simulink model "sixth_harmonic"  (R2013a)
settings: Solver=ode4  StartTime=0.0  StopTime=0.1  FixedStep=Ts  RelTol=1e-3
values from neighbouring files (symbols this model uses):
  Ip1 = Iline_fund*sqrt(2)    [acemp_sixth.m]    (also in immd_simulation_base.m)
  Ip3 = Iline_three*sqrt(2)    [acemp_sixth.m]    (also in immd_simulation_base.m)
  Lload = Xload/wout_fund    [acemp_sixth.m]    (also in immd_base_varyingmod.m = Xload/wout; immd_design_elen.m = Xload/wout; immd_efficiency.m = Xload/wout; immd_simulation_base.m)
  ma1 = 0.8    [acemp_sixth.m]    (also in immd_simulation_base.m)
  ma3 = 0.3    [acemp_sixth.m]    (also in immd_simulation_base.m)
  Rload = Zload*pf    [acemp_sixth.m]    (also in immd_base_varyingmod.m; immd_design_elen.m; immd_efficiency.m; immd_simulation_base.m)
  Ts = 1e-6    (= 1e-06)    [acemp_sixth.m]    (also in immd_base_varyingmod.m = 1e-05; immd_design_elen.m; immd_efficiency.m; immd_simulation_base.m)
  Vdc = (3/pi)*Vs_ll*sqrt(2)    [IMMD_design_tool_v01.m]    (also in IMMD_design_tool_v02.m; acemp_sixth.m = 400; immd_base_varyingmod.m = 400; immd_capacitor_rms_current.m = 400)
  Vp1 = ma1*Vdc/2    (= 160)    [acemp_sixth.m]    (also in immd_simulation_base.m)
  Vp3 = ma3*Vdc/2    (= 60)    [acemp_sixth.m]    (also in immd_simulation_base.m)
  wout_fund = 2*pi*fout_fund    (= 314.159265359)    [acemp_sixth.m]    (also in immd_simulation_base.m)
  wout_three = 2*pi*fout_three    (= 942.477796077)    [acemp_sixth.m]    (also in immd_simulation_base.m)
libraries: powerlib x32, powerlib_meascontrol x14
settings Model: Creator=ugurm  LastModifiedBy=ugurm

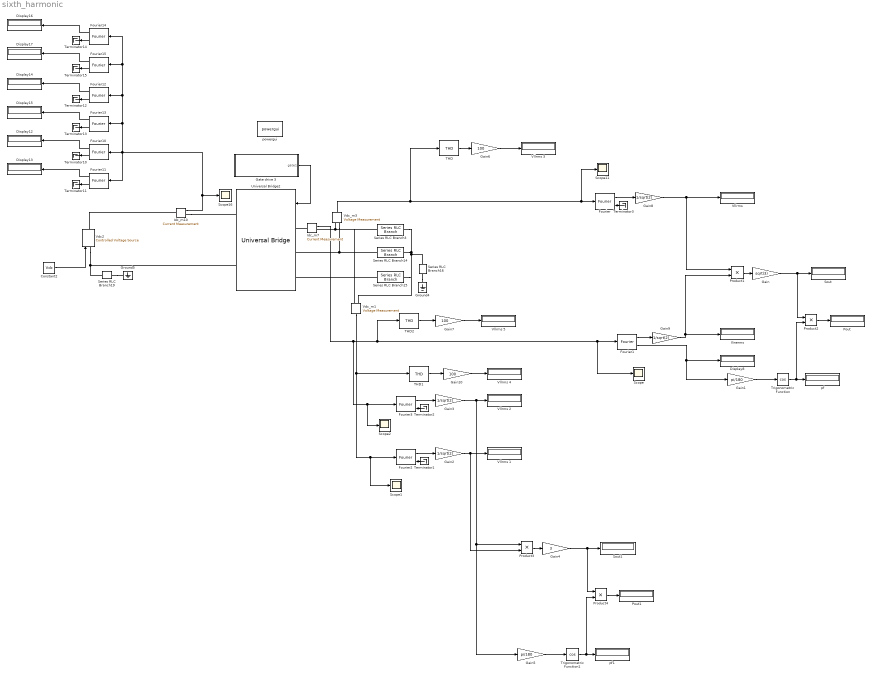
== system sixth_harmonic ==
  Constant2 : Constant  Value=Vdc
  Display{8,12..17} (7 alike) : Display
  Fourier : powerlib_meascontrol/Measurements/Fourier  Freq=fout_fund  n=1  InInit=[0, 0]  Ts=Ts
  Fourier1 : powerlib_meascontrol/Measurements/Fourier  Freq=fout_fund  n=1  InInit=[0, 0]  Ts=Ts
  Fourier10 : powerlib_meascontrol/Measurements/Fourier  Freq=fout_fund  n=1  InInit=[0, 0]  Ts=Ts
  Fourier11 : powerlib_meascontrol/Measurements/Fourier  Freq=fout_fund  n=0  InInit=[0, 0]  Ts=Ts
  Fourier12 : powerlib_meascontrol/Measurements/Fourier  Freq=fout_fund  n=3  InInit=[0, 0]  Ts=Ts
  Fourier13 : powerlib_meascontrol/Measurements/Fourier  Freq=fout_fund  n=2  InInit=[0, 0]  Ts=Ts
  Fourier14 : powerlib_meascontrol/Measurements/Fourier  Freq=fout_fund  n=6  InInit=[0, 0]  Ts=Ts
  Fourier15 : powerlib_meascontrol/Measurements/Fourier  Freq=fout_fund  n=4  InInit=[0, 0]  Ts=Ts
  Fourier2 : powerlib_meascontrol/Measurements/Fourier  Freq=fout_fund  n=3  InInit=[0, 0]  Ts=Ts
  Fourier3 : powerlib_meascontrol/Measurements/Fourier  Freq=fout_fund  n=3  InInit=[0, 0]  Ts=Ts
  Gain : Gain  Gain=sqrt(3)
  Gain1 : Gain  Gain=pi/180
  Gain10 : Gain  Gain=100
  Gain{2..3,8..9} (4 alike) : Gain  Gain=1/sqrt(2)
  Gain4 : Gain  Gain=3
  Gain5 : Gain  Gain=pi/180
  Gain6 : Gain  Gain=100
  Gain7 : Gain  Gain=100
  Gate drive 3 : Subsystem
  Ground4 : powerlib/Elements/Ground  LConnTagsString=a
  Ground5 : powerlib/Elements/Ground  LConnTagsString=a
  Idc_m10 : powerlib/Measurements/Current Measurement  PhasorSimulation=off  OutputType=Complex  PSBequivalent=0
  Idc_m7 : powerlib/Measurements/Current Measurement  PhasorSimulation=off  OutputType=Complex  PSBequivalent=0
  "Ilinerms " : Display
  Pout : Display
  Pout1 : Display
  Product{1..4} (4 alike) : Product
  Scope{,1..2,11,16} (5 alike) : Scope
      Scope settings: YMin=32  YMax=45
      Scope1 settings: YMin=-10  YMax=10  SaveName=vphase
      Scope11 settings: YMin=-400  YMax=400  SaveName=vline
      Scope16 settings: TimeRange=0.05  YMin=0  YMax=8  SaveName=idc3
      Scope2 settings: YMin=-10  YMax=10  SaveName=iline
  Series RLC Branch14 : powerlib/Elements/Series RLC Branch  LConnTagsString=__new0  RConnTagsString=__new0  BranchType=RL  Resistance=Rload  Inductance=Lload  SetiL0=off  InitialCurrent=0  Capacitance=1e-6  Setx0=off  InitialVoltage=0  Measurements=None
  Series RLC Branch15 : powerlib/Elements/Series RLC Branch  LConnTagsString=__new0  RConnTagsString=__new0  BranchType=RL  Resistance=Rload  Inductance=Lload  SetiL0=off  InitialCurrent=0  Capacitance=1e-6  Setx0=off  InitialVoltage=0  Measurements=None
  Series RLC Branch16 : powerlib/Elements/Series RLC Branch  LConnTagsString=__new0  RConnTagsString=__new0  BranchType=R  Resistance=1e12  Inductance=Lload  SetiL0=off  InitialCurrent=0  Capacitance=1e-6  Setx0=off  InitialVoltage=0  Measurements=None
  Series RLC Branch19 : powerlib/Elements/Series RLC Branch  LConnTagsString=__new0  RConnTagsString=__new0  BranchType=R  Resistance=1e12  Inductance=Lload  SetiL0=off  InitialCurrent=0  Capacitance=1e-6  Setx0=off  InitialVoltage=0  Measurements=None
  Series RLC Branch3 : powerlib/Elements/Series RLC Branch  LConnTagsString=__new0  RConnTagsString=__new0  BranchType=RL  Resistance=Rload  Inductance=Lload  SetiL0=off  InitialCurrent=0  Capacitance=1e-6  Setx0=off  InitialVoltage=0  Measurements=None
  Sout : Display
      settings: Format=short_e
  Sout1 : Display
      settings: Format=short_e
  THD : powerlib_meascontrol/Measurements/THD  Freq=fout_fund  Ts=Ts
  THD1 : powerlib_meascontrol/Measurements/THD  Freq=fout_fund  Ts=Ts
  THD2 : powerlib_meascontrol/Measurements/THD  Freq=fout_fund  Ts=Ts
  Terminator{1..3,10..15} (9 alike) : Terminator
  Trigonometric Function : Trigonometry  Operator=cos
  Trigonometric Function1 : Trigonometry  Operator=cos
  Universal Bridge2 : powerlib/Power Electronics/Universal Bridge  Arms=3  SnubberResistance=1e5  SnubberCapacitance=inf  Device=IGBT / Diodes  Ron=1e-6  Lon=0  ForwardVoltages="[  0  0  ]"  ForwardVoltage=0  GTOparameters=[ 10e-6 , 20e-6 ]  IGBTparameters=[0,0]  Measurements=None  Measurements_2=None  converterType=Rectifier
  Vdc2 : powerlib/Electrical Sources/Controlled Voltage Source  Initialize=off  Source_Type=DC  Amplitude=200  Phase=0  Frequency=0  Measurements=None
  Vdc_m1 : powerlib/Measurements/Voltage Measurement  PhasorSimulation=off  OutputType=Complex  PSBequivalent=0
  Vdc_m3 : powerlib/Measurements/Voltage Measurement  PhasorSimulation=off  OutputType=Complex  PSBequivalent=0
  Vllrms {,1..5} (6 alike) : Display
  pf : Display
  pf1 : Display
  powergui : powerlib/powergui  Priority=1  SimulationMode=Discrete  SolverType=Tustin  SampleTime=Ts  frequency=60  SPID=off  DisableSnubberDevices=off  DisableRonSwitches=off  DisableVfSwitches=off  SwTol=0  Interpol=off  DisplayEquations=off  frequencyindice=0  Pbase=100e6  ErrMax=1e-4  Iterations=50  UnitsV=kV  UnitsW=MW  FunctionMessages=off  echomessages=off  HookPort=off  EnableUseOfTLC=off  x0status=blocks  RestoreLinks=warning  ResistiveCurrentMeasurement=off  Frange=[0:2:500]  Ylog=off  Xlog=on  ShowGrid=off  save=off  variable=ZData  structure=ptotal  ZoomFFT=off  StartTime=0.02  cycles=4  DisplayStyle=5  fundamental=50  FreqAxis=off  MaxFrequency=1000  frequencyindicesteady=1  RmsSteady=1  display=off  Ts=0  methode=off
  wires:
  Gate drive 3/1(gate1) -> Universal Bridge2/1
  Vdc_m3/1 -> THD/1, Fourier/1, Scope11/1
  Constant2/1 -> Vdc2/1
  Fourier10/1 -> Display12/1
  Fourier10/2 -> Terminator10/1
  Fourier11/1 -> Display13/1
  Fourier11/2 -> Terminator11/1
  Fourier12/1 -> Display14/1
  Fourier12/2 -> Terminator12/1
  Fourier13/1 -> Display15/1
  Fourier13/2 -> Terminator13/1
  Fourier14/1 -> Display16/1
  Fourier14/2 -> Terminator14/1
  Idc_m10/1 -> Fourier14/1, Fourier15/1, Fourier12/1, Fourier13/1, Fourier11/1, Fourier10/1, Scope16/1
  Fourier15/1 -> Display17/1
  Fourier15/2 -> Terminator15/1
  Gain8/1 -> Product1/1, "Vllrms "/1
  Gain9/1 -> "Ilinerms "/1, Product1/2
  Idc_m7/1 -> Scope2/1, Fourier3/1, THD2/1, Scope/1, Fourier1/1
  Fourier1/1 -> Gain9/1
  Fourier/1 -> Gain8/1
  Product1/1 -> Gain/1
  Gain/1 -> Product2/1, Sout/1
  Fourier1/2 -> Gain1/1, Display8/1
  Trigonometric Function/1 -> Product2/2, pf/1
  Gain1/1 -> Trigonometric Function/1
  Product2/1 -> Pout/1
  Fourier/2 -> Terminator3/1
  Fourier2/1 -> Gain2/1
  Fourier2/2 -> Terminator1/1
  Gain3/1 -> Gain5/1, Product3/1, Vllrms 2/1
  Fourier3/1 -> Gain3/1
  Fourier3/2 -> Terminator2/1
  Product3/1 -> Gain4/1
  Gain4/1 -> Product4/1, Sout1/1
  Trigonometric Function1/1 -> Product4/2, pf1/1
  Gain5/1 -> Trigonometric Function1/1
  Product4/1 -> Pout1/1
  Gain2/1 -> Product3/2, Vllrms 1/1
  Vdc_m1/1 -> THD1/1, Scope1/1, Fourier2/1
  THD/1 -> Gain6/1
  THD1/1 -> Gain10/1
  THD2/1 -> Gain7/1
  Gain6/1 -> Vllrms 3/1
  Gain7/1 -> Vllrms 5/1
  Gain10/1 -> Vllrms 4/1
  connections:
  Vdc_m3/LConn2 -- Series RLC Branch14/LConn1 -- Universal Bridge2/LConn2
  Vdc_m3/LConn1 -- Vdc_m1/LConn1 -- Series RLC Branch3/LConn1 -- Idc_m7/RConn1
  Series RLC Branch14/RConn1 -- Series RLC Branch3/RConn1 -- Vdc_m1/LConn2 -- Series RLC Branch15/RConn1 -- Series RLC Branch16/LConn1
  Idc_m7/LConn1 -- Universal Bridge2/LConn1
  Series RLC Branch16/RConn1 -- Ground4/LConn1
  Series RLC Branch15/LConn1 -- Universal Bridge2/LConn3
  Series RLC Branch19/LConn1 -- Universal Bridge2/RConn2 -- Vdc2/LConn1
  Vdc2/RConn1 -- Idc_m10/LConn1
  Series RLC Branch19/RConn1 -- Ground5/LConn1
  Idc_m10/RConn1 -- Universal Bridge2/RConn1

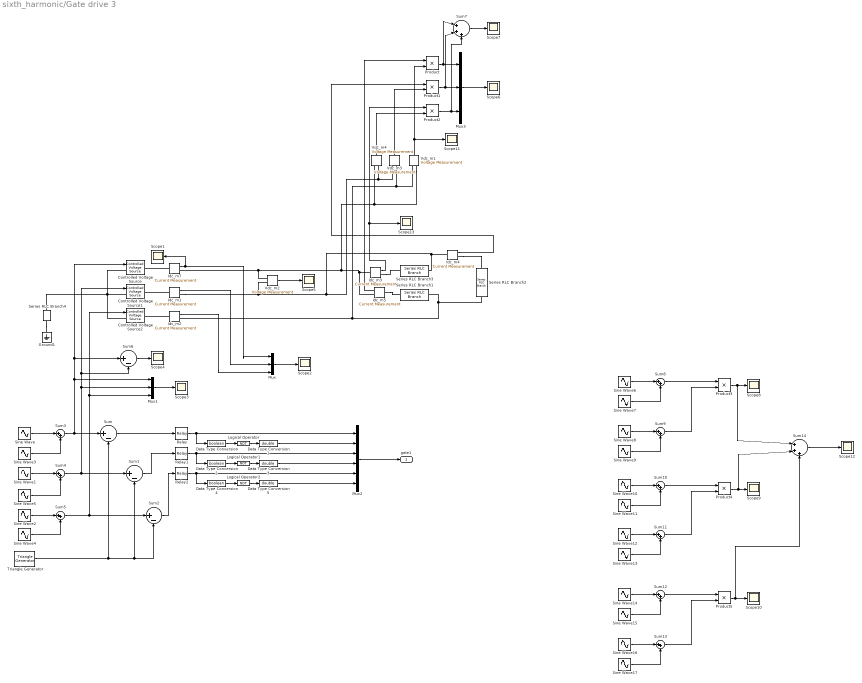
== system sixth_harmonic/Gate drive 3 ==
  Controlled Voltage Source : powerlib/Electrical Sources/Controlled Voltage Source  Initialize=on  Source_Type=AC  Amplitude=0  Phase=0  Frequency=0  Measurements=None
  Controlled Voltage Source1 : powerlib/Electrical Sources/Controlled Voltage Source  Initialize=on  Source_Type=AC  Amplitude=0  Phase=0  Frequency=0  Measurements=None
  Controlled Voltage Source2 : powerlib/Electrical Sources/Controlled Voltage Source  Initialize=on  Source_Type=AC  Amplitude=0  Phase=0  Frequency=0  Measurements=None
  Data Type Conversion : DataTypeConversion  OutDataTypeStr=boolean
  Data Type Conversion1 : DataTypeConversion  OutDataTypeStr=double
  Data Type Conversion2 : DataTypeConversion  OutDataTypeStr=boolean
  Data Type Conversion3 : DataTypeConversion  OutDataTypeStr=double
  Data Type Conversion4 : DataTypeConversion  OutDataTypeStr=boolean
  Data Type Conversion5 : DataTypeConversion  OutDataTypeStr=double
  Ground1 : powerlib/Elements/Ground  LConnTagsString=a
  Idc_m{1..5,7} (6 alike) : powerlib/Measurements/Current Measurement  PhasorSimulation=off  OutputType=Complex  PSBequivalent=0
  Logical Operator : Logic  Operator=NOT  AllPortsSameDT=off  OutDataTypeStr=boolean
  Logical Operator1 : Logic  Operator=NOT  AllPortsSameDT=off  OutDataTypeStr=boolean
  Logical Operator2 : Logic  Operator=NOT  AllPortsSameDT=off  OutDataTypeStr=boolean
  Mux : Mux  Inputs=3
  Mux1 : Mux  Inputs=3
  Mux2 : Mux  Inputs=6
  Mux3 : Mux  Inputs=3
  Product{,1..5} (6 alike) : Product
  Relay : Relay
  Relay1 : Relay
  Relay2 : Relay
  Scope{1..13} (13 alike) : Scope
      Scope1 settings: YMin=-0.25  YMax=0.225  SaveName=vline2
      Scope10 settings: YMin=0  YMax=6500  SaveName=pct
      Scope11 settings: YMin=-1.75  YMax=1  SaveName=vline1
      Scope12 settings: YMin=4000  YMax=19000  SaveName=ptotal
      Scope13 settings: YMin=-1.75  YMax=1  SaveName=vline8
      Scope2 settings: YMin=-0.275  YMax=0.275  SaveName=vline3
      Scope3 settings: YMin=-1.75  YMax=1.75  SaveName=vline4
      Scope4 settings: YMin=-1.75  YMax=1.75  SaveName=vline5
      Scope5 settings: YMin=-1.75  YMax=1.75  SaveName=vline6
      Scope6 settings: YMin=-0.05  YMax=0.9  SaveName=vline7
      Scope7 settings: YMin=0.35  YMax=1  SaveName=power
      Scope8 settings: YMin=0  YMax=6500  SaveName=pat
      Scope9 settings: YMin=0  YMax=6500  SaveName=pbt
  Series RLC Branch1 : powerlib/Elements/Series RLC Branch  LConnTagsString=__new0  RConnTagsString=__new0  BranchType=RL  Resistance=Rload  Inductance=Lload  SetiL0=off  InitialCurrent=0  Capacitance=1e-6  Setx0=off  InitialVoltage=0  Measurements=None
  Series RLC Branch2 : powerlib/Elements/Series RLC Branch  LConnTagsString=__new0  RConnTagsString=__new0  BranchType=RL  Resistance=Rload  Inductance=Lload  SetiL0=off  InitialCurrent=0  Capacitance=1e-6  Setx0=off  InitialVoltage=0  Measurements=None
  Series RLC Branch3 : powerlib/Elements/Series RLC Branch  LConnTagsString=__new0  RConnTagsString=__new0  BranchType=RL  Resistance=Rload  Inductance=Lload  SetiL0=off  InitialCurrent=0  Capacitance=1e-6  Setx0=off  InitialVoltage=0  Measurements=None
  Series RLC Branch4 : powerlib/Elements/Series RLC Branch  LConnTagsString=__new0  RConnTagsString=__new0  BranchType=R  Resistance=1e12  Inductance=Lload  SetiL0=off  InitialCurrent=0  Capacitance=1e-6  Setx0=off  InitialVoltage=0  Measurements=None
  Sine Wave : Sin  Amplitude=ma1  Frequency=wout_fund  SampleTime=0
  Sine Wave1 : Sin  Amplitude=ma1  Frequency=wout_fund  Phase=-2*pi/3  SampleTime=0
  Sine Wave10 : Sin  Amplitude=Vp1  Frequency=wout_fund  Phase=-2*pi/3  SampleTime=0
  Sine Wave11 : Sin  Amplitude=Vp3  Frequency=wout_three  Phase=-2*pi/3  SampleTime=0
  Sine Wave12 : Sin  Amplitude=Ip1  Frequency=wout_fund  Phase=-2*pi/3  SampleTime=0
  Sine Wave13 : Sin  Amplitude=Ip3  Frequency=wout_three  Phase=-2*pi/3  SampleTime=0
  Sine Wave14 : Sin  Amplitude=Vp1  Frequency=wout_fund  Phase=-4*pi/3  SampleTime=0
  Sine Wave15 : Sin  Amplitude=Vp3  Frequency=wout_three  Phase=-4*pi/3  SampleTime=0
  Sine Wave16 : Sin  Amplitude=Ip1  Frequency=wout_fund  Phase=-4*pi/3  SampleTime=0
  Sine Wave17 : Sin  Amplitude=Ip3  Frequency=wout_three  Phase=-4*pi/3  SampleTime=0
  Sine Wave2 : Sin  Amplitude=ma1  Frequency=wout_fund  Phase=2*pi/3  SampleTime=0
  Sine Wave3 : Sin  Amplitude=ma3  Frequency=wout_three  SampleTime=0
  Sine Wave4 : Sin  Amplitude=ma3  Frequency=wout_three  SampleTime=0
  Sine Wave5 : Sin  Amplitude=ma3  Frequency=wout_three  SampleTime=0
  Sine Wave6 : Sin  Amplitude=Vp1  Frequency=wout_fund  SampleTime=0
  Sine Wave7 : Sin  Amplitude=Vp3  Frequency=wout_three  SampleTime=0
  Sine Wave8 : Sin  Amplitude=Ip1  Frequency=wout_fund  SampleTime=0
  Sine Wave9 : Sin  Amplitude=Ip3  Frequency=wout_three  SampleTime=0
  Sum{,1..2,6} (4 alike) : Sum  Inputs=|+-
  Sum{3..5,8..13} (9 alike) : Sum  Inputs=|++
  Sum14 : Sum  Inputs=|+++
  Sum7 : Sum  Inputs=|+++
  Triangle Generator : powerlib_meascontrol/Pulse & Signal Generators/Triangle Generator  Freq=fsw  Phase=0  Ts=Ts
  Vdc_m{1..4} (4 alike) : powerlib/Measurements/Voltage Measurement  PhasorSimulation=off  OutputType=Complex  PSBequivalent=0
  gate1 : Outport
  wires:
  Triangle Generator/1 -> Sum/2, Sum1/2, Sum2/2
  Sum/1 -> Relay/1
  Sum1/1 -> Relay1/1
  Sum2/1 -> Relay2/1
  Data Type Conversion/1 -> Logical Operator/1
  Relay/1 -> Data Type Conversion/1, Mux2/1
  Logical Operator/1 -> Data Type Conversion1/1
  Data Type Conversion1/1 -> Mux2/2
  Data Type Conversion2/1 -> Logical Operator1/1
  Relay1/1 -> Data Type Conversion2/1, Mux2/3
  Logical Operator1/1 -> Data Type Conversion3/1
  Data Type Conversion3/1 -> Mux2/4
  Data Type Conversion4/1 -> Logical Operator2/1
  Relay2/1 -> Data Type Conversion4/1, Mux2/5
  Logical Operator2/1 -> Data Type Conversion5/1
  Data Type Conversion5/1 -> Mux2/6
  Mux2/1 -> gate1/1
  Sine Wave/1 -> Sum3/1
  Sine Wave3/1 -> Sum3/2
  Sum3/1 -> Mux1/1, Sum6/1, Controlled Voltage Source/1, Sum/1
  Sum4/1 -> Mux1/2, Controlled Voltage Source1/1, Sum6/2, Sum1/1
  Sine Wave1/1 -> Sum4/1
  Sine Wave5/1 -> Sum4/2
  Sine Wave2/1 -> Sum5/1
  Sine Wave4/1 -> Sum5/2
  Sum5/1 -> Mux1/3, Controlled Voltage Source2/1, Sum2/1
  Idc_m7/1 -> Mux/1, Scope1/1
  Idc_m1/1 -> Mux/2
  Mux/1 -> Scope2/1
  Mux1/1 -> Scope3/1
  Sum6/1 -> Scope4/1
  Vdc_m2/1 -> Scope5/1
  Vdc_m1/1 -> Product/2, Scope11/1
  Mux3/1 -> Scope6/1
  Product/1 -> Sum7/1, Mux3/1
  Product1/1 -> Sum7/2, Mux3/2
  Product2/1 -> Sum7/3, Mux3/3
  Idc_m2/1 -> Mux/3
  Vdc_m3/1 -> Product1/2
  Vdc_m4/1 -> Product2/2
  Sum7/1 -> Scope7/1
  Sine Wave6/1 -> Sum8/1
  Sine Wave7/1 -> Sum8/2
  Sum8/1 -> Product3/1
  Sine Wave8/1 -> Sum9/1
  Sine Wave9/1 -> Sum9/2
  Sum9/1 -> Product3/2
  Product3/1 -> Sum14/1, Scope8/1
  Sine Wave10/1 -> Sum10/1
  Sine Wave11/1 -> Sum10/2
  Sum10/1 -> Product4/1
  Sine Wave12/1 -> Sum11/1
  Sine Wave13/1 -> Sum11/2
  Sum11/1 -> Product4/2
  Product4/1 -> Sum14/2, Scope9/1
  Sine Wave14/1 -> Sum12/1
  Sine Wave15/1 -> Sum12/2
  Sum12/1 -> Product5/1
  Sine Wave16/1 -> Sum13/1
  Sine Wave17/1 -> Sum13/2
  Sum13/1 -> Product5/2
  Product5/1 -> Sum14/3, Scope10/1
  Sum14/1 -> Scope12/1
  Idc_m3/1 -> Scope13/1, Product2/1
  Idc_m4/1 -> Product1/1
  Idc_m5/1 -> Product/1
  connections:
  Idc_m7/LConn1 -- Controlled Voltage Source/RConn1
  Controlled Voltage Source2/LConn1 -- Controlled Voltage Source/LConn1 -- Series RLC Branch4/LConn1 -- Controlled Voltage Source1/LConn1
  Series RLC Branch4/RConn1 -- Ground1/LConn1
  Idc_m1/LConn1 -- Controlled Voltage Source1/RConn1
  Idc_m1/RConn1 -- Vdc_m2/LConn2 -- Vdc_m3/LConn1 -- Vdc_m4/LConn2 -- Idc_m4/LConn1 -- Series RLC Branch3/RConn1
  Idc_m2/LConn1 -- Controlled Voltage Source2/RConn1
  Series RLC Branch2/RConn1 -- Series RLC Branch1/RConn1 -- Vdc_m1/LConn1 -- Vdc_m3/LConn2 -- Idc_m2/RConn1
  Vdc_m2/LConn1 -- Idc_m5/RConn1 -- Idc_m3/LConn1 -- Vdc_m1/LConn2 -- Vdc_m4/LConn1 -- Idc_m7/RConn1
  Idc_m3/RConn1 -- Series RLC Branch3/LConn1
  Idc_m4/RConn1 -- Series RLC Branch2/LConn1
  Idc_m5/LConn1 -- Series RLC Branch1/LConn1
